simulink model "LQR_PI_2017"  (R2017a)
settings: Solver=ode1  StartTime=0.0  StopTime=30  FixedStep=0.002  RelTol=1e-3  EnableMultiTasking=on
InitFcn:
  | LQR_IntMiah
values from neighbouring files (symbols this model uses):
  K = 1.35*K_hat(1:m,1:n)    [LQR_PI_Int.m]
  Ki = -K_hat(1:m,n+1:n+p)    [LQR_PI_Int.m]
undefined symbols (not defined in the file or in its folder): C
libraries: simulink_extras x5, quarc_library x3, quanser_aero x1
settings Model: SimulationMode=external  ExtModeTrigDuration=10000  Creator=MLevis  LastModifiedBy=kvonckx
settings SolverCC: PositivePriorityOrder=on
settings DataIOCC: LimitDataPoints=on  SaveFormat=Array
settings OptimizationCC: LifeSpan=inf
settings DebuggingCC: SolverPrmCheckMsg=warning  SFUnexpectedBacktrackingDiag=warning  SFNoUnconditionalDefaultTransitionDiag=warning  SFExecutionAtInitializationDiag=none
settings HardwareCC: ProdBitPerPointer=32  ProdBitPerSizeT=32  ProdBitPerPtrDiffT=32  ProdLargestAtomicFloat=None  ProdIntDivRoundTo=Undefined  ProdEndianess=Unspecified  ProdWordSize=32  ProdHWDeviceType=32-bit Generic
settings ModelReferenceCC: PropagateSignalLabelsOutOfModel=off
settings RTWCC: SystemTargetFile=quarc_win64.tlc  TemplateMakefile=quarc_default_tmf  Description=QUARC Win64 Target
settings STFCustomTargetCC: TargetPreCompLibLocation=C:\PROGRA~3\QUARC\lib\2017a\win64\release  ConcurrentExecutionCompliant=on  GeneratePreprocessorConditionals=Disable all  SystemTargetFile=quarc_win64.tlc
settings GRTTargetCC: TargetPreCompLibLocation=C:\PROGRA~3\QUARC\lib\2017a\win64\release  TargetLangStandard=C89/C90 (ANSI)  ParMdlRefBuildCompliant=off  CompOptLevelCompliant=off  GeneratePreprocessorConditionals=Disable all  CombineOutputUpdateFcns=off  MatFileLogging=off  CPPClassGenCompliant=off  GRTInterface=on  UseToolchainInfoCompliant=off  ExtMode=on  ExtModeMexFile=quarc_comm
settings ConfigComp: CovMetricSettings=dw  CovHtmlReporting=on  CovSaveCumulativeToWorkspaceVar=on  CovSaveSingleToWorkspaceVar=on  CovExternalEMLEnable=off  CovSFcnEnable=off

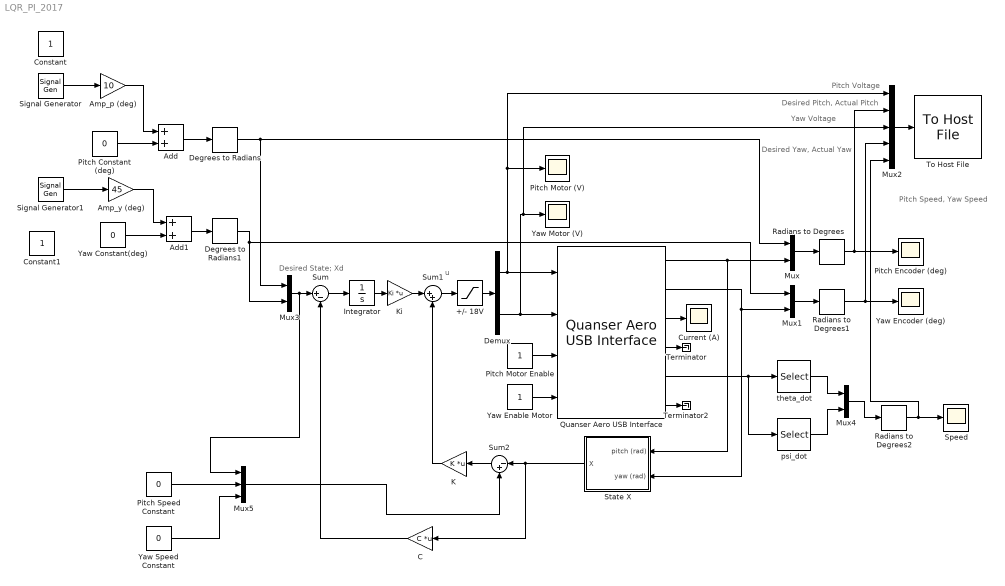
== system LQR_PI_2017 ==
  note: Desired State; Xd
  note: u
  note: Pitch Voltage
  note: Desired Pitch, Actual Pitch
  note: Desired Yaw, Actual Yaw
  note: Yaw Voltage
  note: Pitch Speed, Yaw Speed
  +/- 18V : Saturate  UpperLimit=18  LowerLimit=-18
  Add : Sum
  Add1 : Sum
  Amp_p (deg) : Gain  Gain=10
  Amp_y (deg) : Gain  Gain=45
  "C " : Gain  Gain=C  Multiplication=Matrix(K*u)
  Constant : Constant
  Constant1 : Constant
  Current (A) : Scope
  Degrees to Radians : simulink_extras/Transformations/Degrees to Radians
  Degrees to Radians1 : simulink_extras/Transformations/Degrees to Radians
  Demux : Demux  Outputs=2
  Integrator : Integrator
  K : Gain  Gain=K  Multiplication=Matrix(K*u)
  Ki : Gain  Gain=Ki  Multiplication=Matrix(K*u)
  Mux{,1,3..4} (4 alike) : Mux  Inputs=2
  Mux2 : Mux  Inputs=5
  Mux5 : Mux  Inputs=3
  Pitch Constant (deg) : Constant  Value=0
  Pitch Encoder (deg) : Scope
  Pitch Motor (V) : Scope
  Pitch Motor Enable : Constant
  Pitch Speed Constant : Constant  Value=0
  Quanser Aero USB Interface : quanser_aero/Quanser Aero USB Interface  SystemSampleTime=-1
  Radians to Degrees : simulink_extras/Transformations/Radians to Degrees
  Radians to Degrees1 : simulink_extras/Transformations/Radians to Degrees
  Radians to Degrees2 : simulink_extras/Transformations/Radians to Degrees
  Signal Generator : SignalGenerator  WaveForm=square  Frequency=0.1
  Signal Generator1 : SignalGenerator  WaveForm=square  Frequency=0.04
  Speed : Scope
  State X : Subsystem
  Sum : Sum  Inputs=|+-
  Sum1 : Sum  Inputs=|++
  Sum2 : Sum  Inputs=|-+
  Terminator : Terminator
  Terminator2 : Terminator
  To Host File : quarc_library/Sinks/To Host/To Host File  file_name=RMSE_LQR_NEW.mat  variable_name=RMSE_LQR_NEW  decimation=1  sample_time=-1  file_format=MAT-file v.4  options=No header or footer  append=off  final_file_name=RMSE_LQR_NEW.mat  bitrate=2000000
  Yaw Constant(deg) : Constant  Value=0
  Yaw Enable Motor : Constant
  Yaw Encoder (deg) : Scope
  Yaw Motor (V) : Scope
  Yaw Speed Constant : Constant  Value=0
  psi_dot : Selector  InputPortWidth=3  IndexOptions=Index vector (dialog)  Indices=[3]  OutputSizes=1
  theta_dot : Selector  InputPortWidth=3  IndexOptions=Index vector (dialog)  Indices=[2]  OutputSizes=1
  wires:
  Degrees to Radians/1 -> Mux3/1, Mux/1
  Degrees to Radians1/1 -> Mux3/2, Mux1/1
  Pitch Constant (deg)/1 -> Add/2
  Add/1 -> Degrees to Radians/1
  Yaw Constant(deg)/1 -> Add1/2
  Amp_p (deg)/1 -> Add/1
  Amp_y (deg)/1 -> Add1/1
  Add1/1 -> Degrees to Radians1/1
  Mux/1 -> Radians to Degrees/1
  Radians to Degrees/1 -> Mux2/2, Pitch Encoder (deg)/1
  Radians to Degrees1/1 -> Yaw Encoder (deg)/1, Mux2/4
  Pitch Motor Enable/1 -> Quanser Aero USB Interface/3
  Yaw Enable Motor/1 -> Quanser Aero USB Interface/4
  Demux/1 -> Quanser Aero USB Interface/1, Mux2/1, Pitch Motor (V)/1
  Demux/2 -> Quanser Aero USB Interface/2, Mux2/3, Yaw Motor (V)/1
  Mux1/1 -> Radians to Degrees1/1
  +/- 18V/1 -> Demux/1
  Quanser Aero USB Interface/3 -> Current (A)/1
  Quanser Aero USB Interface/1 -> Mux/2, State X/1(pitch (rad))
  Quanser Aero USB Interface/2 -> Mux1/2, State X/2(yaw (rad))
  Quanser Aero USB Interface/4 -> Terminator/1
  Quanser Aero USB Interface/6 -> Terminator2/1
  Mux2/1 -> To Host File/1
  Quanser Aero USB Interface/5 -> psi_dot/1, theta_dot/1
  theta_dot/1 -> Mux4/1
  psi_dot/1 -> Mux4/2
  Mux4/1 -> Radians to Degrees2/1
  Radians to Degrees2/1 -> Speed/1, Mux2/5
  State X/1(X) -> Sum2/1, "C "/1
  Ki/1 -> Sum1/1
  Sum1/1 -> +/- 18V/1
  K/1 -> Sum1/2
  "C "/1 -> Sum/2
  Sum/1 -> Integrator/1
  Integrator/1 -> Ki/1
  Sum2/1 -> K/1
  Yaw Speed Constant/1 -> Mux5/3
  Pitch Speed Constant/1 -> Mux5/2
  Mux3/1 -> Mux5/1, Sum/1
  Mux5/1 -> Sum2/2
  Signal Generator/1 -> Amp_p (deg)/1
  Signal Generator1/1 -> Amp_y (deg)/1

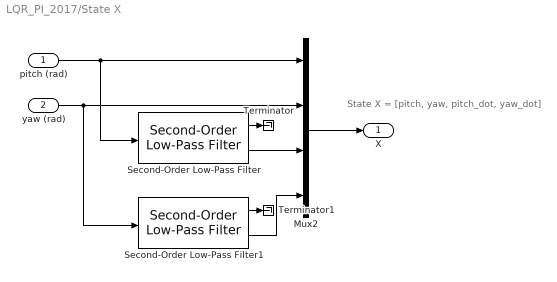
== system LQR_PI_2017/State X ==
  note: State X = [pitch, yaw, pitch_dot, yaw_dot]
  pitch (rad) : Inport
  yaw (rad) : Inport  Port=2
  Mux2 : Mux
  Second-Order Low-Pass Filter : quarc_library/Continuous/Second-Order Low-Pass Filter  params_source=Internal (dialog parameters)  input_width=50  input_zeta=0.8  input_init=0
  Second-Order Low-Pass Filter1 : quarc_library/Continuous/Second-Order Low-Pass Filter  params_source=Internal (dialog parameters)  input_width=50  input_zeta=0.8  input_init=0
  Terminator : Terminator
  Terminator1 : Terminator
  X : Outport
  wires:
  Mux2/1 -> X/1
  yaw (rad)/1 -> Second-Order Low-Pass Filter1/1, Mux2/2
  pitch (rad)/1 -> Second-Order Low-Pass Filter/1, Mux2/1
  Second-Order Low-Pass Filter/2 -> Mux2/3
  Second-Order Low-Pass Filter1/2 -> Mux2/4
  Second-Order Low-Pass Filter/1 -> Terminator/1
  Second-Order Low-Pass Filter1/1 -> Terminator1/1
